simulink model "Electrical787"  (R2013a)
settings: Solver=ode45  StartTime=0.0  StopTime=MSSN.gen.time(end)  RelTol=1e-3
InitFcn:
  | load('SampleOutput.mat')
  | 
  | load('SampleFuelBurn.mat')
undefined symbols (not defined in the file): ailerons, B_737, elevator, FuelBurn, landing_gear, rudder, thrust_rev
libraries: PowerFlowLib x95, simulink x17
(part 1 of 17)
settings Model: Creator=mwillms4  LastModifiedBy=Andrew
settings DataIOCC: SignalLoggingSaveFormat=ModelDataLogs
settings OptimizationCC: ExpressionDepthLimit=2147483647
settings DebuggingCC: FcnCallInpInsideContextMsg=EnableAllAsWarning  UnconnectedInputMsg=none  UnconnectedOutputMsg=none  UnconnectedLineMsg=none
settings GRTTargetCC: CombineOutputUpdateFcns=off  GRTInterface=on

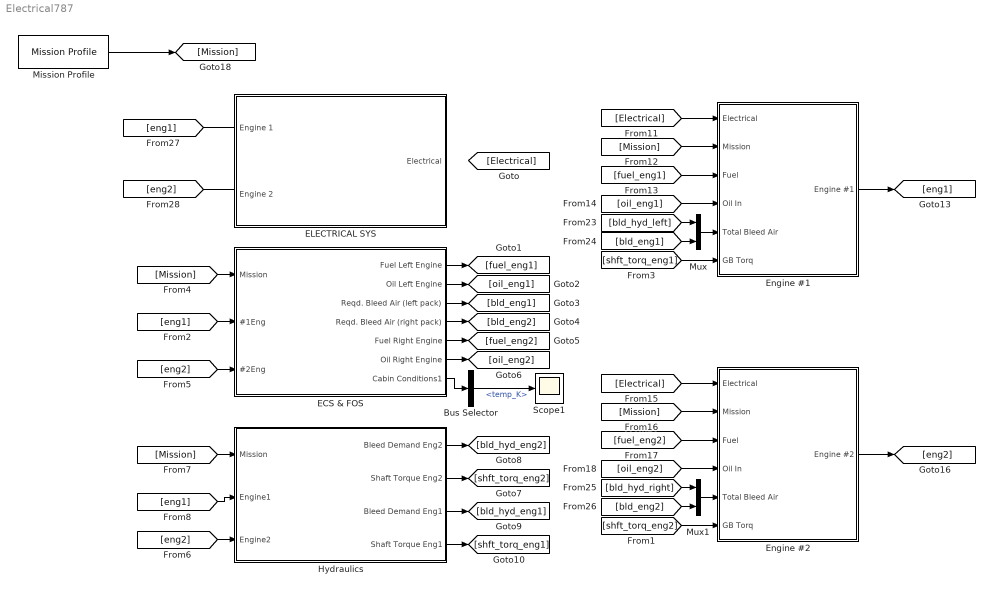
== system Electrical787 ==
  Bus Selector : BusSelector  OutputSignals=temp_K
  "ECS & FOS " : Subsystem
  "ELECTRICAL SYS " : Subsystem
  Engine #1 : Subsystem
  Engine #2 : Subsystem
  "Hydraulics " : Subsystem
  Mission Profile : PowerFlowLib/Mission Profile/Mission Profile  mssn_check=off  mssn_prof=MSSN  del_P=0  del_T=0  del_rho=0  pres_msl=101.3  temp_msl=15  dens_msl=1.229
  Mux : Mux  Inputs=2
  Mux1 : Mux  Inputs=2
  Scope1 : Scope
      settings: YMin=282  YMax=299  SaveName=ScopeData36
  wires:
  Mission Profile/1 -> [Mission]
  ? -> [Electrical]
  Engine #1/1(Engine #1) -> [eng1]
  Engine #2/1(Engine #2) -> [eng2]
  "Hydraulics "/1(Bleed Demand Eng2) -> [bld_hyd_eng2]
  "Hydraulics "/3(Bleed Demand Eng1) -> [bld_hyd_eng1]
  "ECS & FOS "/1("Fuel Left Engine ") -> [fuel_eng1]
  "ECS & FOS "/2(Oil Left Engine) -> [oil_eng1]
  "ECS & FOS "/3(Reqd. Bleed Air (left pack)) -> [bld_eng1]
  "ECS & FOS "/4(Reqd. Bleed Air (right pack)) -> [bld_eng2]
  "ECS & FOS "/5(Fuel Right Engine) -> [fuel_eng2]
  "ECS & FOS "/6(Oil Right Engine) -> [oil_eng2]
  [Mission] -> "Hydraulics "/1(Mission)
  [eng2] -> "Hydraulics "/3(Engine2)
  [eng1] -> "Hydraulics "/2(Engine1)
  [Mission] -> "ECS & FOS "/1(Mission)
  [Electrical] -> Engine #1/1(Electrical)
  [Mission] -> Engine #1/2(Mission)
  [fuel_eng1] -> Engine #1/3(Fuel)
  [oil_eng1] -> Engine #1/4(Oil In)
  [Electrical] -> Engine #2/1(Electrical)
  [Mission] -> Engine #2/2(Mission)
  [fuel_eng2] -> Engine #2/3(Fuel)
  [oil_eng2] -> Engine #2/4(Oil In)
  Mux/1 -> Engine #1/5(Total Bleed Air)
  [bld_eng1] -> Mux/2
  [bld_hyd_left] -> Mux/1
  Mux1/1 -> Engine #2/5(Total Bleed Air)
  [bld_eng2] -> Mux1/2
  [bld_hyd_right] -> Mux1/1
  Bus Selector/1 -> Scope1/1  "<temp_K>"
  [eng1] -> "ECS & FOS "/2(#1Eng)
  [eng2] -> "ECS & FOS "/3(#2Eng)
  [eng1] -> ?
  [eng2] -> ?
  "ECS & FOS "/7(Cabin Conditions1) -> Bus Selector/1
  "Hydraulics "/2(Shaft Torque Eng2) -> [shft_torq_eng2]
  "Hydraulics "/4(Shaft Torque Eng1) -> [shft_torq_eng1]
  [shft_torq_eng2] -> Engine #2/6(GB Torq)
  [shft_torq_eng1] -> Engine #1/6(GB Torq)

== system Electrical787/ECS & FOS  ==
  note: Environmental Control System
  note: Fuel & Oil System
  Mission : Inport
  #1Eng : Inport  Port=2
  #2Eng : Inport  Port=3
  #1Eng1 : InportShadow  Port=2
  #1Eng2 : InportShadow  Port=2
  #2Eng1 : InportShadow  Port=3
  #2Eng2 : InportShadow  Port=3
  Bus Creator : BusCreator  Inputs=3
  Bus Selector : BusSelector  OutputSignals=Flight parameters.temp_K,Flight parameters.Mach
  Bus Selector1 : BusSelector  OutputSignals=power_kW
  Cabin Zone : PowerFlowLib/Energy & Power Systems/Thermal/ECS/Cabin Zone  A_fuselage=320  V_cab=130.3  n_pass=176  L_shell=0.003  K_shell=1  L_insulation=0.02  K_insulation=1  L_coating=0.002  K_coating=1  Vdot_sa_pass=0.009438  q_pass=60  RAR=.25  h_outside=1  h_inside=1
  Constant : Constant  Value=50
  Constant1 : Constant  Value=1700
  Constant2 : Constant  Value=1700
  Constant{3..6} (4 alike) : Constant  Value=0
  ElectricalSink : PowerFlowLib/Support Functions//Tools/ElectricalSink  Tag=Flow  Description=TwoPhase  load_loc=Empennage  ACDC_load=AC  units=Kilowatts  unq_id=6691
  ElectricalSink1 : PowerFlowLib/Support Functions//Tools/ElectricalSink  Tag=Flow  Description=TwoPhase  load_loc=Cagobay  ACDC_load=AC  units=Kilowatts  unq_id=1878
  ElectricalSink2 : PowerFlowLib/Support Functions//Tools/ElectricalSink  Tag=Flow  Description=TwoPhase  load_loc=Cabin  ACDC_load=AC  units=Kilowatts  unq_id=3506
  ElectricalSink4 : PowerFlowLib/Support Functions//Tools/ElectricalSink  Tag=Flow  Description=TwoPhase  load_loc=Cabin  ACDC_load=DC  units=Kilowatts  unq_id=8332
  Fan1 : PowerFlowLib/Energy & Power Systems/Thermal/ECS/Fan  N_fan=1725
  Fuel Tanks/Pumps : Subsystem
  Heat Exchanger : PowerFlowLib/Energy & Power Systems/Thermal/Fuel & Oil/Heat Exchanger  fld1=Oil  fld2=Air  Tw_init=90  C_wall=60000  Tw0=90  Q0=20000  H1_0=10000  A1=0.18984  mdot1_0=1.2  Tin1_0=105  Pin1_0=101  H2_0=10000  A2=0.045127  mdot2_0=1  Tin2_0=35  Pin2_0=50
  Heat Exchanger1 : PowerFlowLib/Energy & Power Systems/Thermal/Fuel & Oil/Heat Exchanger  fld1=Oil  fld2=Air  Tw_init=90  C_wall=60000  Tw0=90  Q0=20000  H1_0=10000  A1=0.18984  mdot1_0=1.2  Tin1_0=105  Pin1_0=101  H2_0=10000  A2=0.045127  mdot2_0=1  Tin2_0=35  Pin2_0=50
  Heat Exchanger2 : PowerFlowLib/Energy & Power Systems/Thermal/Fuel & Oil/Heat Exchanger  fld1=Oil  fld2=Fuel  Tw_init=80  C_wall=60000  Tw0=80  Q0=40000  H1_0=20000  A1=0.17164  mdot1_0=1  Tin1_0=55  Pin1_0=100  H2_0=20000  A2=0.53191  mdot2_0=1.2  Tin2_0=95  Pin2_0=101
  Heat Exchanger3 : PowerFlowLib/Energy & Power Systems/Thermal/Fuel & Oil/Heat Exchanger  fld1=Fuel  fld2=Oil  Tw_init=80  C_wall=60000  Tw0=80  Q0=40000  H1_0=20000  A1=0.53191  mdot1_0=1.2  Tin1_0=95  Pin1_0=101  H2_0=20000  A2=0.17164  mdot2_0=1  Tin2_0=55  Pin2_0=100
  Left PACK : Subsystem
  Memory : Memory
  Mission1 : InportShadow
  Oil Tanks/Pumps Left Wing : Subsystem
  Oil Tanks/Pumps Left Wing1 : Subsystem
  Right PACK : Subsystem
  Thermal_sources_from Electrical_power_model1 : Subsystem
  n-intlet Mixing Junction : PowerFlowLib/Energy & Power Systems/Thermal/ECS/n-intlet Mixing Junction  no_inlets=3  d_in_1=0.1  d_in_2=0.1  d_out=0.2
  "Fuel Left Engine " : Outport
  Oil Left Engine : Outport  Port=2
  Reqd. Bleed Air (left pack) : Outport  Port=3
  Reqd. Bleed Air (right pack) : Outport  Port=4
  Fuel Right Engine : Outport  Port=5
  Oil Right Engine : Outport  Port=6
  Cabin Conditions1 : Outport  Port=7
  wires:
  Left PACK/1(Reqd. Bleed air) -> Reqd. Bleed Air (left pack)/1
  Mission/1 -> Left PACK/2(MISSION), Right PACK/2(MISSION)
  Right PACK/2(Reqd. Bleed air) -> Reqd. Bleed Air (right pack)/1
  Constant/1 -> Fuel Tanks/Pumps/1(Pamb)
  Heat Exchanger1/1 -> Heat Exchanger3/2
  Fuel Tanks/Pumps/2(Fuel Right Wing) -> Heat Exchanger3/1
  Oil Tanks/Pumps Left Wing1/1(Oil To HX) -> Heat Exchanger1/1
  Constant1/1 -> Oil Tanks/Pumps Left Wing1/1(Oil Sys Pres)
  Heat Exchanger3/1 -> Fuel Right Engine/1
  Heat Exchanger/1 -> Heat Exchanger2/1
  Oil Tanks/Pumps Left Wing/1(Oil To HX) -> Heat Exchanger/1
  Constant2/1 -> Oil Tanks/Pumps Left Wing/1(Oil Sys Pres)
  Fuel Tanks/Pumps/1(Fuel Left Wing) -> Heat Exchanger2/2
  Heat Exchanger2/2 -> "Fuel Left Engine "/1
  Heat Exchanger3/2 -> Oil Right Engine/1
  Constant3/1 -> ElectricalSink1/1, ElectricalSink2/1, ElectricalSink2/2, ElectricalSink1/2, ElectricalSink/1, ElectricalSink/2
  n-intlet Mixing Junction/1 -> Memory/1
  Mission1/1 -> Bus Selector/1
  Bus Selector/1 -> Cabin Zone/2  "<temp_K>"
  Bus Selector/2 -> Cabin Zone/3  "<Mach>"
  Thermal_sources_from Electrical_power_model1/1(Thermal Loads) -> Cabin Zone/4
  Left PACK/2(Flow Out) -> n-intlet Mixing Junction/2
  Memory/1 -> Cabin Zone/1
  #1Eng2/1 -> Oil Tanks/Pumps Left Wing/2(Flow In)
  #2Eng1/1 -> Fuel Tanks/Pumps/2(Fuel Demand Right Wing)
  #1Eng1/1 -> Fuel Tanks/Pumps/3(Fuel Demand Left Wing)
  #2Eng/1 -> Oil Tanks/Pumps Left Wing1/2(Flow In)
  #1Eng/1 -> Left PACK/1(ENGINE)
  #2Eng2/1 -> Right PACK/1(ENGINE)
  Cabin Zone/1 -> Cabin Conditions1/1, [Cabin_conditions]
  [Fan_Mixing_Jn] -> n-intlet Mixing Junction/1
  [Cabin_conditions] -> Right PACK/3(Cabin Conditions)
  [Cabin_conditions] -> Left PACK/3(Cabin Conditions)
  Right PACK/1(Flow Out) -> n-intlet Mixing Junction/3
  Bus Selector1/1 -> ElectricalSink4/1  "<power_kW>"
  Cabin Zone/2 -> Fan1/1
  Fan1/1 -> [Fan_Mixing_Jn]
  Fan1/2 -> Bus Selector1/1
  Heat Exchanger2/1 -> Oil Left Engine/1
  Bus Creator/1 -> Heat Exchanger1/2, Heat Exchanger/2
  Constant4/1 -> Bus Creator/1  "pres_kPa"
  Constant5/1 -> Bus Creator/2  "temp_K"
  Constant6/1 -> Bus Creator/3  "mdot_kgps"

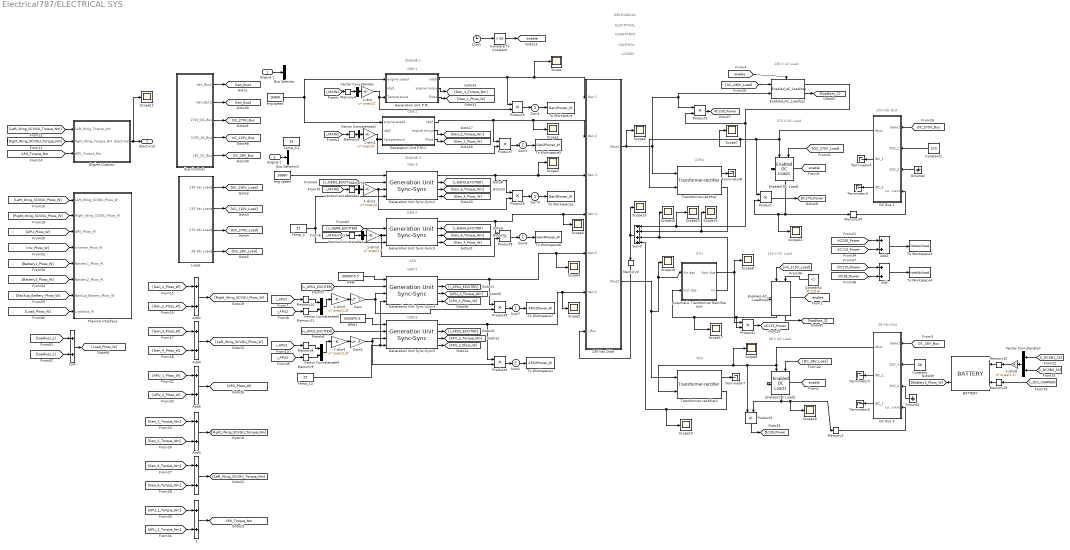
== system Electrical787/ELECTRICAL SYS  ==
  note: GEN 1
  note: ENGINE 1
  note: GEN 2
  note: GEN 3
  note: ENGINE 2
  note: GEN 4
  note: GEN 5
  note: APU
  note: GEN 6
  note: ATRU
  note: TRU
  note: 230 V AC Load
  note: 270 Vdc Dist
  note: 28 Vdc Dist
  note: 270 V DC Load
  note: CONSTANTS
  note: CONTROL
  note: LOSSES
  note: MECHANICAL
  note: ELECTRICAL
  note: ATU
  note: 115 V AC Load
  note: 28 V DC Load
  Engine 1 : Inport
  Engine 2 : Inport  Port=2
  " " : Sum
  " 1" : Sum
  1-dim{,1..3} (4 alike) : Gain  Gain=ones(1)'  Multiplication=Matrix(u*K)
  1-dim4 : Gain  Gain=ones(1,2)'  Multiplication=Matrix(u*K)
  1-dim5 : Gain  Gain=ones(1,2)'  Multiplication=Matrix(u*K)
  1-dim8 : Gain  Gain=ones(1,2)'  Multiplication=Matrix(u*K)
  230 Vac Distr : Subsystem
  Add{,1..5} (6 alike) : Sum
  Automatic Transformer Rectifier Unit : Subsystem
  BATTERY : PowerFlowLib/Energy & Power Systems/Electrical/Battery/BATTERY  NO_CELLS=9  NO_MODULES=10  INITIAL_SOC=1
  Bus Selector : BusSelector  OutputSignals=Spools.HPSpoolSpeed_rpm
  Bus Selector1 : BusSelector  OutputSignals=Spools.HPSpoolSpeed_rpm
  Bus Controls : Subsystem  mask{BUS1=Generator 1, BUS2=Generator 2, MBUS1=Generator Bus 1, ACTBUS1=Generator Bus 1, MBUS2=Generator Bus 2, ACTBUS2=Generator Bus 2, IDCBUS1=Battery 1, IDCBUS2=Battery 2}
      mask prompts: BUS1 "Source for Bus 1"; BUS2 "Source for Bus 2"; MBUS1 "Load on Main Bus 1 drawn from"; ACTBUS1 "Load on AC Transfer Bus 1 drawn from"; MBUS2 "Load on Main Bus 2 drawn from"; ACTBUS2 "Load on AC Transfer Bus 2 drawn from"; IDCBUS1 "Source for DC Service Bus 1"; IDCBUS2 "Source for DC Service Bus 2"
      mask help:
      | Specify the source from which different buses receive power. There are
      | 1. Two Generator buses (Bus 1-2)
      | 2. Two AC Main buses (Main Bus 1-2))
      | 3. Two AC Transfer buses and (AC Transfer Bus 1-2)
      | 4. Two DC Intermediate buses (DC Intermediate Bus 1-2)
      mask init:
      | switch BUS1
      |     case 1
      |         BUS1CONTROL = 1;
      |     case 2
      |         BUS1CONTROL = 2;
      |     case 3
      |         BUS1CONTROL = 3;
      |     case 4
      |         BUS1CONTROL = 4;
      | end
      | 
      | switch BUS2
      |     case 1
      |         BUS2CONTROL = 1;
      |     case 2
      |         BUS2CONTROL = 2;
      |     case 3
      |         BUS2CONTROL = 3;
      |     case 4
      |         BUS2CONTROL = 4;
      | end
      | 
      | switch MBUS1
      |     case 1
      |         MBUS1CONTROL = 1;
      |     case 2
      |         MBUS1CONTROL = 2;
      | end
      | 
      | switch ACTBUS1
      |     case 1
      |         ACTBUS1CONTROL = 1;
      |     case 2
      |         ACTBUS1CONTROL = 2;
      | end
      | 
      | switch MBUS2
      |     case 1
      |         MBUS2CONTROL = 1;
      |     case 2
      |         MBUS2CONTROL = 2;
      | end
      | 
      | switch ACTBUS2
      |     case 1
      |         ACTBUS2CONTROL = 1;
      |     case 2
      |         ACTBUS2CONTROL = 2;
      | end
      | 
      | switch IDCBUS1
      |     case 1
      |         IDCBUS1CONTROL = 1;
      |     case 2
      |         IDCBUS1CONTROL = 2;
      | end
      | 
      | switch IDCBUS2
      |     case 1
      |         IDCBUS2CONTROL = 1;
      |     case 2
      |         IDCBUS2CONTROL = 2;
      | end
      mask TypeOptions BUS1: Generator 1  | APU  | GND | AUX SUPPLY
      mask TypeOptions BUS2: Generator 2  | APU  | GND | AUX SUPPLY
      mask TypeOptions MBUS1: Generator Bus 1 | Generator Bus 2
      mask TypeOptions ACTBUS1: Generator Bus 1 | Generator Bus 2
      mask TypeOptions MBUS2: Generator Bus 1 | Generator Bus 2
      mask TypeOptions ACTBUS2: Generator Bus 1 | Generator Bus 2
      mask TypeOptions IDCBUS1: Battery 1 | Battery 2
      mask TypeOptions IDCBUS2: Battery 1 | Battery 2
  Clock : Clock
  Compare To Constant : simulink/Logic and Bit Operations/Compare To Constant  relop=>  const=50  OutDataTypeStr=uint8
  Constant : Constant  Value=28
  Constant1 : Constant  Value=270
  Constant2 : Constant  Value=[0,115,0]
  DC Bus 1 : Subsystem  mask(DC Service Bus){}
      mask help: Service Bus
  DC Bus 3 : Subsystem  mask(DC Service Bus){}
      mask help: Service Bus
  Enabled DC Load1 : PowerFlowLib/Energy & Power Systems/Electrical/Loads/Enabled  DC Load1
  Enabled DC Load2 : PowerFlowLib/Energy & Power Systems/Electrical/Loads/Enabled  DC Load1
  Enabled_AC_Loadloss : PowerFlowLib/Energy & Power Systems/Electrical/Loads/Enabled_AC_Loadloss  P=500  PF=0.85  ILRMS=0  R=10000  X=10000
  Enabled_AC_Loadloss1 : PowerFlowLib/Energy & Power Systems/Electrical/Loads/Enabled_AC_Loadloss  P=500  PF=0.85  ILRMS=0  R=10000  X=10000
  Engine Outputs : Subsystem
  Gain : Gain  Gain=.5  Multiplication=Matrix(u*K)
  Gain1 : Gain  Gain=.5  Multiplication=Matrix(u*K)
  Generation Unit P.M. : Subsystem  AncestorBlock=PowerFlowLib/Energy & Power Systems/Electrical/Systems/Generation Unit Sync-Sync  mask{machine_mode=100kVA_Gen, Rs=0.0163, Xls=0.00054, Xmd=0.66176, Xmq=0.00099, R_fd=0.016, Xlfd=0.2092, R_1d=0.2047, Xl1d=0.6524, R_1q=0.0429, R_2q=0.0429, Xl1q=0.0639, Xl2q=0.0639, ws=377, RTL=0.001, XTL=0.1, KA=20, KF=0.063, T_f=0.35, TA=0.2, KE=1, TE=0.314, SB=100000, VBDQ=100, wB=377, P=6, H=0.1777, R_conv_gen=0.05, mc_gen=10000, Vnom=230, fan_load='init_fan_characteristics.mat', exciter_param='exciter.mat'}
      mask prompts: machine_mode "Machine Preset"; Rs "Stator Resistance [ohm]"; Xls "Stator Leakage Reactance [ohm]"; Xmd "Magnetizing Direct Axis Reactance [ohm]"; Xmq "Magnetizing Quadrature Axis Reactance [ohm]"; R_fd "Field Resistance [ohm]"; Xlfd "Field Leakage Reactance [ohm]"; R_1d "Transient Direct Axis Resistance [ohm]"; Xl1d "Transient Leakage Direct Axis Reactance [ohm]"; R_1q "Transient Quadrature Axis Resistance [ohm]"; R_2q "Subtransient Quadrature Axis Resistance [ohm]"; Xl1q "Transient Leakage Quadrature Axis Reactance [ohm]"; Xl2q "Subtransient Leakage Quadrature Axis Reactance [ohm]"; ws "Rotational Speed [rad/s]"; RTL "Resistance [ohm]"; XTL "Reactance [ohm]"; SB "Baes Complex Power [VA]"; VBDQ "Base Direct and Quadrature Axis Armature Voltage [V]"; wB "Base Electrical Frequency [rad/s]"; P "Number of Pole Pairs"; H "Shaft Inertia Constant [s]"; Vnom "Nominal Voltage [V]"; fan_load "Fan Load"; exciter_param "Exciter Machine Parameters"
      mask help:
      | A generator system block implements a generic power generation unit consisting of a gearbox, a synchronous generator, a synchronous exciter and exciter controls.
      | The generator size can be selected from the drop window below.
      | (For advanced-users) When the User-defined option is selected from the drop window, the generator parameters can be manually specified in the tabs below.
      |
      | Block Inputs:
      |
      | #1: Jet engine low pressure spool [RPM]
      | #2: Exciter system supply voltage [V]
      | #3: Synchronous reference frame line currents  [A]
      |
      | Block Output:
      |
      | #1: Synchronous reference frame line voltages [V]
      | #2: Exciter system supply current [A]
      | #3: Electromagnetic torque on the low pressure spool  [N-M]
      | #4: Heat rejected to the cooling system or ambient [W]
      mask init:
      | load(fan_load);
      | 
      | % Inductances
      | Xd = Xls + Xmd;
      | Xq = Xls + Xmq;
      | Xfd = Xlfd + Xmd;
      | X1q = Xl1q + Xmq;
      | Xd1 = Xd - Xmd^2/Xfd;
      | Xq1 = Xq - Xmq^2/X1q;
      | Xd2 = Xls + (1/(1/Xmd + 1/Xlfd + 1/Xl1d));
      | Xq2 = Xls + (1/(1/Xmq + 1/Xl1q + 1/Xl2q));
      | Tdo1 = Xfd/ws/R_fd;
      | Tqo1 = X1q/ws/R_1q;
      | Tdo2 = 1/ws/R_1d*(Xl1d + 1/(1/Xmd + 1/Xlfd));
      | Tqo2 = 1/ws/R_2q*(Xl2q+1/(1/Xmq + 1/Xl1q));
      | 
      | % Base Quantities
      | 
      | TB = (P/2)*SB/wB;
      | IBDQ = SB/VBDQ;
      | LBDQ = VBDQ/wB;
      | 
      | IBFD = IBDQ;
      | IB1D = IBDQ;
      | IB1Q = IBDQ;
      | IB2Q = IBDQ;
      | 
      | VBFD = SB/IBFD;
      | VB1D = SB/IB1D;
      | VB1Q = SB/IB1Q;
      | VB2Q = SB/IB2Q;
      | 
      | LBFD = VBFD/wB;
      | LB1D = VB1D/wB;
      | LB1Q = VB1Q/wB;
      | LB2Q = VB2Q/wB;
      | 
      | J = 2*H/(wB*2/P)^2*SB;
      | M = 2*H/wB;
      | 
      | % Exciter
      | 
      | data_exc = load(exciter_param);
      |   
      | % Stator
      | Rs_exc = data_exc.r(1);
      | Xls_exc = data_exc.r(2);
      | Xmd_exc = data_exc.r(3);
      | Xmq_exc = data_exc.r(4);
      | 
      | % Field
      | R_fd_exc = data_exc.r(5);
      | Xlfd_exc = data_exc.r(6);
      | % Dampers
      | R_1d_exc = data_exc.r(7);
      | Xl1d_exc = data_exc.r(8);
      | R_1q_exc = data_exc.r(9);
      | Xl1q_exc = data_exc.r(10);
      | R_2q_exc = data_exc.r(11);
      | Xl2q_exc = data_exc.r(12);
      | 
      | % Rotor
      | P_exc = data_exc.r(13);
      | ws_exc = data_exc.r(14);
      | 
      | % Inductances
      | Xd_exc = Xls_exc + Xmd_exc;
      | Xq_exc = Xls_exc + Xmq_exc;
      | Xfd_exc = Xlfd_exc + Xmd_exc;
      | X1q_exc = Xl1q_exc + Xmq_exc;
      | Xd1_exc = Xd_exc - Xmd_exc^2/Xfd_exc;
      | Xq1_exc = Xq_exc - Xmq_exc^2/X1q_exc;
      | Xd2_exc = Xls_exc + (1/(1/Xmd_exc + 1/Xlfd_exc + 1/Xl1d_exc));
      | Xq2_exc = Xls_exc + (1/(1/Xmq_exc + 1/Xl1q_exc + 1/Xl2q_exc));
      | Tdo1_exc = Xfd_exc/ws_exc/R_fd_exc;
      | Tqo1_exc = X1q_exc/ws_exc/R_1q_exc;
      | Tdo2_exc = 1/ws_exc/R_1d_exc*(Xl1d_exc + 1/(1/Xmd_exc + 1/Xlfd_exc));
      | Tqo2_exc = 1/ws_exc/R_2q_exc*(Xl2q_exc+1/(1/Xmq_exc + 1/Xl1q_exc));
      | 
      | % Transmission Line
      | RTL_exc = data_exc.r(15);
      | XTL_exc = data_exc.r(16);
      | 
      | % Regulator and Governor
      | KA_exc = data_exc.r(17);
      | KF_exc = data_exc.r(18);
      | T_f_exc = data_exc.r(19);
      | TA_exc = data_exc.r(20);
      | KE_exc = data_exc.r(21);
      | TE_exc = data_exc.r(22);
      | 
      | % Base Quantities
      | SB_exc = data_exc.r(23);
      | VBDQ_exc = data_exc.r(24);
      | wB_exc = data_exc.r(25);
      | P_exc = data_exc.r(13);
      | H_exc = data_exc.r(26);
      | 
      | TB_exc = (P/2)*SB_exc/wB_exc;
      | IBDQ_exc = SB_exc/VBDQ_exc;
      | LBDQ_exc = VBDQ_exc/wB_exc;
      | 
      | IBFD_exc = IBDQ_exc;
      | IB1D_exc = IBDQ_exc;
      | IB1Q_exc = IBDQ_exc;
      | IB2Q_exc = IBDQ_exc;
      | 
      | VBFD_exc = SB_exc/IBFD_exc;
      | VB1D_exc = SB_exc/IB1D_exc;
      | VB1Q_exc = SB_exc/IB1Q_exc;
      | VB2Q_exc = SB_exc/IB2Q_exc;
      | 
      | LBFD_exc = VBFD_exc/wB_exc;
      | LB1D_exc = VB1D_exc/wB_exc;
      | LB1Q_exc = VB1Q_exc/wB_exc;
      | LB2Q_exc = VB2Q_exc/wB_exc;
      | 
      | J_exc = 2*data_exc.r(26)/(wB_exc*2/P_exc)^2*SB_exc;
      | M_exc = 2*H_exc/wB_exc;
      | 
      | R_conv_gen_exc = 1/data_exc.r(27);
      | mc_gen_exc = data_exc.r(28);
      mask Help: eval('open(''Generator System_help.html'')');
      mask TypeOptions machine_mode: 20kVA_Gen | 52.5kVA_Gen | 100kVA_Gen | 300kVA_Gen | 800kVA_Gen | 1MVA_Gen | User-defined
      mask Callback machine_mode:
      | h=get_param(gcb,'handle');
      | hblock=get(h);
      | data=load('GenProp.mat');
      | 
      | if strcmp(hblock.machine_mode,'User-defined')==1;
      |     adv_warn=warndlg(sprintf('User-defined parameters may lead to an unstable build.'));
      | 
      |     % grabs current values of enabled GUI parameters
      |     mskenabl = get_param(gcb,'MaskEnables');
      |     mskenabl(1:size(mskenabl,1)) = {'on'};  % sets all parameters to enable
      |     set_param(gcb,'MaskEnables',mskenabl)
      | 
      | else
      |     % For each generator preset references a column from GenProp.mat
      |     if strcmp(hblock.machine_mode,'20kVA_Gen')==1; n=1;
      |     elseif strcmp(hblock.machine_mode,'52.5kVA_Gen')==1; n=2;
      |     elseif strcmp(hblock.machine_mode,'100kVA_Gen')==1; n=3;
      |     elseif strcmp(hblock.machine_mode,'300kVA_Gen')==1; n=4;
      |     elseif strcmp(hblock.machine_mode,'800kVA_Gen')==1; n=5;
      |     elseif strcmp(hblock.machine_mode,'1MVA_Gen')==1; n=6;
      |     end
      |     % Set each parameter of the generator
      |     set1=num2str(data.r(1,n));
      |     set2=num2str(data.r(2,n));
      |     set3=num2str(data.r(3,n));
      |     set4=num2str(data.r(4,n));
      |     set_param(gcb,'Rs',set1,'Xls',set2,'Xmd',set3,'Xmq',set4)
      |     set1=num2str(data.r(5,n));
      |     set2=num2str(data.r(6,n));
      |     set_param(gcb,'R_fd',set1,'Xlfd',set2) %5 and 6
      |     set1=num2str(data.r(7,n));
      |     set2=num2str(data.r(8,n));
      |     set3=num2str(data.r(9,n));
      |     set4=num2str(data.r(10,n));
      |     set5=num2str(data.r(11,n));
      |     set6=num2str(data.r(12,n));
      |     set_param(gcb,'R_1d',set1,'Xl1d',set2,'R_1q',set3,'Xl1q',set4,'R_2q',set5,'Xl2q',set6) %7-12
      |     set1=num2str(data.r(14,n));
      |     set2=num2str(data.r(15,n));
      |     set3=num2str(data.r(16,n));
      |     set_param(gcb,'ws',set1,'RTL',set2,'XTL',set3)
      |     set1=num2str(data.r(17,n));
      |     set2=num2str(data.r(18,n));
      |     set3=num2str(data.r(19,n));
      |     set4=num2str(data.r(20,n));
      |     set5=num2str(data.r(21,n));
      |     set6=num2str(data.r(22,n));
      |     set_param(gcb,'KA',set1,'KF',set2,'T_f',set3,'TA',set4,'KE',set5,'TE',set6)
      |     set1=num2str(data.r(23,n));
      |     set2=num2str(data.r(24,n));
      |     set3=num2str(data.r(25,n));
      |     set4=num2str(data.r(13,n));
      |     set5=num2str(data.r(26,n));
      |     set_param(gcb,'SB',set1,'VBDQ',set2,'wB',set3,'P',set4,'H',set5)
      |     set1=num2str(1/data.r(27,n));
      |     set2=num2str(data.r(28,n));
      |     set_param(gcb,'R_conv_gen',set1,'mc_gen',set2)
      | 
      |     % grabs current values of enabled GUI parameters
      |     mskenabl = get_param(gcb,'MaskEnables');
      |     % sets all parameters to enable
      |     mskenabl(2:size(mskenabl,1)-3) = {'off'};
      |     set_param(gcb,'MaskEnables',mskenabl)
      | 
      | 
      | end
      | 
      | 
      | clear h hblock n data mskenabl
      | clear set1 set2 set3 set4 set5 set6
      mask Display:
      | image(imread('Generator.png')) % Load image
      | 
      | % Define inputs
      | 
      | port_label('input',1,'{\bf \omega_s_h_a_f_t}','Texmode','on')
      | port_label('input',2,'{\bf V_D_C}','Texmode','on')
      | port_label('input',3,'{\bf I_d_q_0}','Texmode','on')
      | port_label('input',4,'{\bf Temp}','Texmode','on')
      | 
      | % Define outputs
      | 
      | port_label('output',1,'{\bf V_d_q_0}','Texmode','on')
      | port_label('output',2,'{\bf I_D_C}','Texmode','on')
      | port_label('output',3,'{\bf \tau}','Texmode','on')
      | port_label('output',4,'{\bf P_l_o_s_s}','Texmode','on')
      | 
      | % % Define inputs
      | %
      | % port_label('input',1,'{\bf Generator Speed}','Texmode','on')
      | % port_label('input',2,'{\bf Battery Voltage}','Texmode','on')
      | % port_label('input',3,'{\bf Line Currents}','Texmode','on')
      | %
      | % % Define outputs
      | %
      | % port_label('output',1,'{\bf Line Voltages}','Texmode','on')
      | % port_label('output',2,'{\bf Battery Current}','Texmode','on')
      | % port_label('output',3,'{\bf Generator Torque}','Texmode','on')
      | % port_label('output',4,'{\bf Power Loss}','Texmode','on')
  Generation Unit P.M.1 : Subsystem  AncestorBlock=PowerFlowLib/Energy & Power Systems/Electrical/Systems/Generation Unit Sync-Sync  mask{machine_mode=100kVA_Gen, Rs=0.0163, Xls=0.00054, Xmd=0.66176, Xmq=0.00099, R_fd=0.016, Xlfd=0.2092, R_1d=0.2047, Xl1d=0.6524, R_1q=0.0429, R_2q=0.0429, Xl1q=0.0639, Xl2q=0.0639, ws=377, RTL=0.001, XTL=0.1, KA=20, KF=0.063, T_f=0.35, TA=0.2, KE=1, TE=0.314, SB=100000, VBDQ=100, wB=377, P=6, H=0.1777, R_conv_gen=0.05, mc_gen=10000, Vnom=230, fan_load='init_fan_characteristics.mat', exciter_param='exciter.mat'}
      mask prompts: machine_mode "Machine Preset"; Rs "Stator Resistance [ohm]"; Xls "Stator Leakage Reactance [ohm]"; Xmd "Magnetizing Direct Axis Reactance [ohm]"; Xmq "Magnetizing Quadrature Axis Reactance [ohm]"; R_fd "Field Resistance [ohm]"; Xlfd "Field Leakage Reactance [ohm]"; R_1d "Transient Direct Axis Resistance [ohm]"; Xl1d "Transient Leakage Direct Axis Reactance [ohm]"; R_1q "Transient Quadrature Axis Resistance [ohm]"; R_2q "Subtransient Quadrature Axis Resistance [ohm]"; Xl1q "Transient Leakage Quadrature Axis Reactance [ohm]"; Xl2q "Subtransient Leakage Quadrature Axis Reactance [ohm]"; ws "Rotational Speed [rad/s]"; RTL "Resistance [ohm]"; XTL "Reactance [ohm]"; SB "Baes Complex Power [VA]"; VBDQ "Base Direct and Quadrature Axis Armature Voltage [V]"; wB "Base Electrical Frequency [rad/s]"; P "Number of Pole Pairs"; H "Shaft Inertia Constant [s]"; Vnom "Nominal Voltage [V]"; fan_load "Fan Load"; exciter_param "Exciter Machine Parameters"
      mask help:
      | A generator system block implements a generic power generation unit consisting of a gearbox, a synchronous generator, a synchronous exciter and exciter controls.
      | The generator size can be selected from the drop window below.
      | (For advanced-users) When the User-defined option is selected from the drop window, the generator parameters can be manually specified in the tabs below.
      |
      | Block Inputs:
      |
      | #1: Jet engine low pressure spool [RPM]
      | #2: Exciter system supply voltage [V]
      | #3: Synchronous reference frame line currents  [A]
      |
      | Block Output:
      |
      | #1: Synchronous reference frame line voltages [V]
      | #2: Exciter system supply current [A]
      | #3: Electromagnetic torque on the low pressure spool  [N-M]
      | #4: Heat rejected to the cooling system or ambient [W]
      mask init: same as Electrical787/ELECTRICAL SYS /Generation Unit P.M.
      mask Help: eval('open(''Generator System_help.html'')');
      mask TypeOptions machine_mode: 20kVA_Gen | 52.5kVA_Gen | 100kVA_Gen | 300kVA_Gen | 800kVA_Gen | 1MVA_Gen | User-defined
      mask Callback machine_mode:
      | h=get_param(gcb,'handle');
      | hblock=get(h);
      | data=load('GenProp.mat');
      | 
      | if strcmp(hblock.machine_mode,'User-defined')==1;
      |     adv_warn=warndlg(sprintf('User-defined parameters may lead to an unstable build.'));
      | 
      |     % grabs current values of enabled GUI parameters
      |     mskenabl = get_param(gcb,'MaskEnables');
      |     mskenabl(1:size(mskenabl,1)) = {'on'};  % sets all parameters to enable
      |     set_param(gcb,'MaskEnables',mskenabl)
      | 
      | else
      |     % For each generator preset references a column from GenProp.mat
      |     if strcmp(hblock.machine_mode,'20kVA_Gen')==1; n=1;
      |     elseif strcmp(hblock.machine_mode,'52.5kVA_Gen')==1; n=2;
      |     elseif strcmp(hblock.machine_mode,'100kVA_Gen')==1; n=3;
      |     elseif strcmp(hblock.machine_mode,'300kVA_Gen')==1; n=4;
      |     elseif strcmp(hblock.machine_mode,'800kVA_Gen')==1; n=5;
      |     elseif strcmp(hblock.machine_mode,'1MVA_Gen')==1; n=6;
      |     end
      |     % Set each parameter of the generator
      |     set1=num2str(data.r(1,n));
      |     set2=num2str(data.r(2,n));
      |     set3=num2str(data.r(3,n));
      |     set4=num2str(data.r(4,n));
      |     set_param(gcb,'Rs',set1,'Xls',set2,'Xmd',set3,'Xmq',set4)
      |     set1=num2str(data.r(5,n));
      |     set2=num2str(data.r(6,n));
      |     set_param(gcb,'R_fd',set1,'Xlfd',set2) %5 and 6
      |     set1=num2str(data.r(7,n));
      |     set2=num2str(data.r(8,n));
      |     set3=num2str(data.r(9,n));
      |     set4=num2str(data.r(10,n));
      |     set5=num2str(data.r(11,n));
      |     set6=num2str(data.r(12,n));
      |     set_param(gcb,'R_1d',set1,'Xl1d',set2,'R_1q',set3,'Xl1q',set4,'R_2q',set5,'Xl2q',set6) %7-12
      |     set1=num2str(data.r(14,n));
      |     set2=num2str(data.r(15,n));
      |     set3=num2str(data.r(16,n));
      |     set_param(gcb,'ws',set1,'RTL',set2,'XTL',set3)
      |     set1=num2str(data.r(17,n));
      |     set2=num2str(data.r(18,n));
      |     set3=num2str(data.r(19,n));
      |     set4=num2str(data.r(20,n));
      |     set5=num2str(data.r(21,n));
      |     set6=num2str(data.r(22,n));
      |     set_param(gcb,'KA',set1,'KF',set2,'T_f',set3,'TA',set4,'KE',set5,'TE',set6)
      |     set1=num2str(data.r(23,n));
      |     set2=num2str(data.r(24,n));
      |     set3=num2str(data.r(25,n));
      |     set4=num2str(data.r(13,n));
      |     set5=num2str(data.r(26,n));
      |     set_param(gcb,'SB',set1,'VBDQ',set2,'wB',set3,'P',set4,'H',set5)
      |     set1=num2str(1/data.r(27,n));
      |     set2=num2str(data.r(28,n));
      |     set_param(gcb,'R_conv_gen',set1,'mc_gen',set2)
      | 
      |     % grabs current values of enabled GUI parameters
      |     mskenabl = get_param(gcb,'MaskEnables');
      |     % sets all parameters to enable
      |     mskenabl(2:size(mskenabl,1)-3) = {'off'};
      |     set_param(gcb,'MaskEnables',mskenabl)
      | 
      | 
      | end
      | 
      | 
      | clear h hblock n data mskenabl
      | clear set1 set2 set3 set4 set5 set6
      mask Display:
      | image(imread('Generator.png')) % Load image
      | 
      | % Define inputs
      | 
      | port_label('input',1,'{\bf \omega_s_h_a_f_t}','Texmode','on')
      | port_label('input',2,'{\bf V_D_C}','Texmode','on')
      | port_label('input',3,'{\bf I_d_q_0}','Texmode','on')
      | port_label('input',4,'{\bf Temp}','Texmode','on')
      | 
      | % Define outputs
      | 
      | port_label('output',1,'{\bf V_d_q_0}','Texmode','on')
      | port_label('output',2,'{\bf I_D_C}','Texmode','on')
      | port_label('output',3,'{\bf \tau}','Texmode','on')
      | port_label('output',4,'{\bf P_l_o_s_s}','Texmode','on')
      | 
      | % % Define inputs
      | %
      | % port_label('input',1,'{\bf Generator Speed}','Texmode','on')
      | % port_label('input',2,'{\bf Battery Voltage}','Texmode','on')
      | % port_label('input',3,'{\bf Line Currents}','Texmode','on')
      | %
      | % % Define outputs
      | %
      | % port_label('output',1,'{\bf Line Voltages}','Texmode','on')
      | % port_label('output',2,'{\bf Battery Current}','Texmode','on')
      | % port_label('output',3,'{\bf Generator Torque}','Texmode','on')
      | % port_label('output',4,'{\bf Power Loss}','Texmode','on')
  Generation Unit Sync-Sync{2..5} (4 alike) : PowerFlowLib/Energy & Power Systems/Electrical/Systems/Generation Unit Sync-Sync  machine_mode=100kVA_Gen  Rs=0.0163  Xls=0.00054  Xmd=0.66176  Xmq=0.00099  R_fd=0.016  Xlfd=0.2092  R_1d=0.2047  Xl1d=0.6524  R_1q=0.0429  R_2q=0.0429  Xl1q=0.0639  Xl2q=0.0639  ws=377  RTL=0.001  XTL=0.1  KA=20  KF=0.063  T_f=0.35  TA=0.2  KE=1  TE=0.314  SB=100000  VBDQ=100  wB=377  P=6  H=0.1777  R_conv_gen=0.05  mc_gen=10000  Vnom=115  fan_load='init_fan_characteristics.mat'  exciter_param='exciter.mat'
  Ground1 : Ground
  Ground2 : Ground
  Loads : Subsystem
  Memory{2..11,24,29,32} (13 alike) : Memory
  Product{,1..9} (10 alike) : Product
  RPM : Constant  Value=30000*0.5
  RPM1 : Constant  Value=30000*0.5
  Scope{,1..19} (20 alike) : Scope
      Scope settings: ShowLegends=on
      Scope1 settings: ShowLegends=on
      Scope10 settings: ShowLegends=on  SaveName=ScopeData10
      Scope11 settings: ShowLegends=on  SaveName=ScopeData11
      Scope12 settings: ShowLegends=on  SaveName=ScopeData12
      Scope13 settings: ShowLegends=on  SaveName=ScopeData13
      Scope14 settings: ShowLegends=on  SaveName=ScopeData14
      Scope15 settings: ShowLegends=on  SaveName=ScopeData15
      Scope16 settings: ShowLegends=on  SaveName=ScopeData16
      Scope17 settings: ShowLegends=on  SaveName=ScopeData17
      Scope18 settings: ShowLegends=on  SaveName=ScopeData18
      Scope19 settings: ShowLegends=on  SaveName=ScopeData19
      Scope2 settings: ShowLegends=on  SaveName=ScopeData2
      Scope3 settings: ShowLegends=on  SaveName=ScopeData3
      Scope4 settings: ShowLegends=on  SaveName=ScopeData4
      Scope5 settings: ShowLegends=on  SaveName=ScopeData5
      Scope6 settings: ShowLegends=on  SaveName=ScopeData6
      Scope7 settings: ShowLegends=on  SaveName=ScopeData7
      Scope8 settings: ShowLegends=on  SaveName=ScopeData8
      Scope9 settings: ShowLegends=on  SaveName=ScopeData9
  Sum : Sum
  Sum{1..2,4..7} (6 alike) : Sum  Inputs=+
  Sum3 : Sum  Inputs=++++
  Temp_C : Constant  Value=25
  Temp_C1 : Constant  Value=25
  Temp_C2 : Constant  Value=25
  Terminator{3..8} (6 alike) : Terminator
  Thermal Interface : Subsystem
  To Workspace : ToWorkspace  VariableName=Gen1Power_W  SampleTime=10  SaveFormat=Structure With Time
  To Workspace1 : ToWorkspace  VariableName=APU2Power_W  SampleTime=10  SaveFormat=Structure With Time
  To Workspace2 : ToWorkspace  VariableName=Gen3Power_W  SampleTime=10  SaveFormat=Structure With Time
  To Workspace3 : ToWorkspace  VariableName=totalacload  SampleTime=-1  SaveFormat=Timeseries
  To Workspace4 : ToWorkspace  VariableName=totaldcload  SampleTime=-1  SaveFormat=Timeseries
  To Workspace5 : ToWorkspace  VariableName=Gen2Power_W  SampleTime=10  SaveFormat=Structure With Time
  To Workspace6 : ToWorkspace  VariableName=Gen4Power_W  SampleTime=10  SaveFormat=Structure With Time
  To Workspace7 : ToWorkspace  VariableName=APU1Power_W  SampleTime=10  SaveFormat=Structure With Time
  Transformer-rectifier : PowerFlowLib/Energy & Power Systems/Electrical/Systems/Transformer-rectifier  pu=1
  Transformer-rectifier2 : PowerFlowLib/Energy & Power Systems/Electrical/Systems/Transformer-rectifier  pu=1
  Vector Concatenate{,1..3} (4 alike) : Concatenate  NumInputs=1  Mode=Multidimensional array  ConcatenateDimension=2
  Vector Concatenate4 : Concatenate  Mode=Multidimensional array  ConcatenateDimension=2
  Vector Concatenate5 : Concatenate  Mode=Multidimensional array  ConcatenateDimension=2
  Vector Concatenate7 : Concatenate  Mode=Multidimensional array  ConcatenateDimension=2
  eng speed : Constant  Value=16860
  "eng speed " : Constant  Value=16860
  Electrical : Outport
  tag scope: AC115_Power=global, AC230_Power=global, AC_115V_Bus=global, APU_Torque_Nm=global, DC270_Power=global, DC28_Power=global, DC_270V_Bus=global, DC_28V_Bus=global, Gen_Bus1=global, Gen_Bus2=global, enable=global
  wires:
  Generation Unit P.M./1(vdq0) -> Product5/1, Scope/1, 230 Vac Distr/1(Gen 1)
  Generation Unit P.M.1/1(vdq0) -> Product7/1, Scope1/1, 230 Vac Distr/2(Gen 2)
  Generation Unit Sync-Sync2/1 -> Product6/1, Scope2/1, 230 Vac Distr/3(Gen 3)
  Generation Unit Sync-Sync3/1 -> Product8/1, Scope3/1, 230 Vac Distr/4(Gen 4)
  Generation Unit Sync-Sync4/1 -> Product9/1, Scope4/1, 230 Vac Distr/5(Gen 5)
  Generation Unit Sync-Sync5/1 -> Product4/1, Scope5/1, 230 Vac Distr/6(Gen 6)
  230 Vac Distr/1(Vbus1) -> Scope6/1, Enabled_AC_Loadloss/2, Product3/1, Transformer-rectifier/1
  230 Vac Distr/2(Vbus2) -> Transformer-rectifier2/1, Scope10/1, Automatic Transformer Rectifier Unit/1(Vin dqo)
  [enable] -> Enabled_AC_Loadloss/Enable
  DC Bus 1/1(Vbus) -> Scope7/1, Transformer-rectifier/2, Product/1, Enabled DC Load1/1
  DC Bus 3/1(Vbus) -> Enabled DC Load2/1, Product2/1, Scope9/1, Transformer-rectifier2/2
  Enabled DC Load1/1 -> Scope12/1, Product/2, Memory24/1
  Memory24/1 -> DC Bus 1/4(Load current)
  Enabled DC Load2/1 -> Product2/2, Scope18/1, Memory2/1
  Memory2/1 -> DC Bus 3/4(Load current)
  [enable] -> Enabled DC Load1/Enable
  [enable] -> Enabled_AC_Loadloss1/Enable
  [enable] -> Enabled DC Load2/Enable
  Transformer-rectifier2/2 -> Scope19/1, Sum3/4
  Transformer-rectifier/2 -> Sum3/2, Scope15/1
  Enabled_AC_Loadloss/1 -> Product3/2, Scope14/1, Sum3/1
  Sum3/1 -> Scope13/1, Memory3/1
  Memory3/1 -> 230 Vac Distr/7(I_Bus)
  Enabled_AC_Loadloss1/1 -> Scope17/1, Automatic Transformer Rectifier Unit/2(Iout dqo), Product1/2
  Memory32/1 -> BATTERY/1
  1-dim8/1 -> Memory32/1
  [i_DCSB1_S2] -> Vector Concatenate7/1
  [i_DCSB2_S2] -> Vector Concatenate7/2
  Vector Concatenate7/1 -> 1-dim8/1
  Memory29/1 -> BATTERY/2
  [i_DC2_CHARGER] -> Memory29/1
  [AC_230V_Load] -> Enabled_AC_Loadloss/1
  Enabled_AC_Loadloss/2 -> [loadloss_1]
  Add/1 -> To Workspace4/1
  Add1/1 -> To Workspace3/1
  Enabled_AC_Loadloss1/2 -> [loadloss_2]
  [AC_115V_Load] -> Enabled_AC_Loadloss1/1
  [DC_270V_Load] -> Enabled DC Load1/2
  Loads/1(230 Vac Loads) -> [AC_230V_Load]
  Loads/2(115 Vac Loads) -> [AC_115V_Load]
  Loads/3(270 Vdc Loads) -> [DC_270V_Load]
  Loads/4(28 Vdc Loads) -> [DC_28V_Load]
  [DC_270V_Bus] -> DC Bus 1/1(Select)
  [DC_28V_Bus] -> DC Bus 3/1(Select)
  Bus Controls/1(Gen_Bus1) -> [Gen_Bus1]
  Bus Controls/2(Gen_Bus2) -> [Gen_Bus2]
  Bus Controls/5(28V_DC_Bus) -> [DC_28V_Bus]
  BATTERY/2 -> [Battery2_Ploss_W]
  Bus Controls/4(115V_AC_Bus) -> [AC_115V_Bus]
  Bus Controls/3(270V_DC_Bus) -> [DC_270V_Bus]
  [i_MAIN1] -> Memory4/1
  [i_MAIN2] -> Memory6/1
  [i_MAIN2] -> Memory7/1
  [i_MAIN1] -> Memory5/1
  Memory7/1 -> Vector Concatenate3/1
  Vector Concatenate3/1 -> 1-dim3/1
  1-dim3/1 -> Product8/2, Generation Unit Sync-Sync3/3
  Memory6/1 -> Vector Concatenate2/1
  Vector Concatenate2/1 -> 1-dim2/1
  1-dim2/1 -> Product6/2, Generation Unit Sync-Sync2/3
  Memory5/1 -> Vector Concatenate1/1
  Vector Concatenate1/1 -> 1-dim1/1
  1-dim1/1 -> Product7/2, Generation Unit P.M.1/3(Temperature)
  Memory4/1 -> Vector Concatenate/1
  Vector Concatenate/1 -> 1-dim/1
  1-dim/1 -> Generation Unit P.M./3(Temperature), Product5/2
  Clock/1 -> Compare To Constant/1
  Compare To Constant/1 -> [enable]
  Engine 2/1 -> Bus Selector1/1
  Generation Unit Sync-Sync2/2 -> [i_GEN3_EXCITER]
  Generation Unit Sync-Sync3/2 -> [i_GEN4_EXCITER]
  [v_GEN3_EXCITER] -> Generation Unit Sync-Sync2/2
  [v_GEN4_EXCITER] -> Generation Unit Sync-Sync3/2
  Temp_C/1 -> Generation Unit Sync-Sync3/4, Generation Unit Sync-Sync2/4
  Product4/1 -> Sum2/1
  Sum2/1 -> To Workspace1/1
  Vector Concatenate4/1 -> 1-dim4/1
  [i_APU2] -> Memory9/1
  [i_APU1] -> Memory8/1
  Memory8/1 -> Vector Concatenate4/1
  Memory9/1 -> Vector Concatenate4/2
  [v_APU2_EXCITER] -> Generation Unit Sync-Sync5/2
  Temp_C2/1 -> Generation Unit Sync-Sync4/4, Generation Unit Sync-Sync5/4
  Vector Concatenate5/1 -> 1-dim5/1
  [i_APU2] -> Memory11/1
  [i_APU1] -> Memory10/1
  Memory10/1 -> Vector Concatenate5/1
  Memory11/1 -> Vector Concatenate5/2
  [v_APU1_EXCITER] -> Generation Unit Sync-Sync4/2
  Product5/1 -> Sum1/1
  Sum1/1 -> To Workspace/1
  Product6/1 -> Sum4/1
  Sum4/1 -> To Workspace2/1
  Product7/1 -> Sum5/1
  Sum5/1 -> To Workspace5/1
  Product8/1 -> Sum6/1
  Sum6/1 -> To Workspace6/1
  Product9/1 -> Sum7/1
  Sum7/1 -> To Workspace7/1
  [Left_Wing_SCVGU_Torque_Nm] -> Engine Outputs/1(Left_Wing_Toqrue_Nm)
  [Right_Wing_SCVGU_Torque_Nm] -> Engine Outputs/2(Rght_Wing_Torque_Nm)
  [APU_Torque_Nm] -> Engine Outputs/3(APU_Torque_Nm)
  [Left_Wing_SCVGU_Ploss_W] -> Thermal Interface/1(Left_Wing_SCVGU_Ploss_W)
  [Right_Wing_SCVGU_Ploss_W] -> Thermal Interface/2(Right_Wing_SCVGU_Ploss_W)
  [APU_Ploss_W] -> Thermal Interface/3(APU_Ploss_W)
  [Inv_Ploss_W] -> Thermal Interface/4(Inverter_Ploss_W)
  [Battery1_Ploss_W] -> Thermal Interface/5(Battery1_Ploss_W)
  [Battery2_Ploss_W] -> Thermal Interface/6(Battery2_Ploss_W)
  [Backup_Battery_Ploss_W] -> Thermal Interface/7(Backup_Battery_Ploss_W)
  [Load_Ploss_W] -> Thermal Interface/8(Loadloss_W)
  [loadloss_1] -> Sum/1
  [loadloss_2] -> Sum/2
  Sum/1 -> [Load_Ploss_W]
  Generation Unit Sync-Sync4/3 -> [APU_1_Torque_Nm]
  Generation Unit Sync-Sync5/3 -> [APU_2_Torque_Nm]
  Generation Unit Sync-Sync4/2 -> [i_APU1_EXCITER]
  Generation Unit Sync-Sync4/4 -> [APU_1_Ploss_W]
  Generation Unit Sync-Sync5/4 -> [APU_2_Ploss_W]
  Generation Unit Sync-Sync5/2 -> [i_APU2_EXCITER]
  Generation Unit P.M./3(Ploss) -> [Gen_1_Ploss_W]
  Generation Unit P.M./2(engine torque) -> [Gen_1_Torque_Nm]
  Generation Unit P.M.1/2(engine torque) -> [Gen_2_Torque_Nm]
  Generation Unit P.M.1/3(Ploss) -> [Gen_2_Ploss_W]
  Add4/1 -> [Left_Wing_SCVGU_Ploss_W]
  Add2/1 -> [Right_Wing_SCVGU_Ploss_W]
  [Gen_1_Ploss_W] -> Add2/1
  [Gen_2_Ploss_W] -> Add2/2
  Generation Unit Sync-Sync3/4 -> [Gen_4_Ploss_W]
  Generation Unit Sync-Sync2/4 -> [Gen_3_Ploss_W]
  [Gen_4_Ploss_W] -> Add4/2
  [Gen_3_Ploss_W] -> Add4/1
  Add3/1 -> [Right_Wing_SCVGU_Torque_Nm]
  " "/1 -> [Left_Wing_SCVGU_Torque_Nm]
  Generation Unit Sync-Sync3/3 -> [Gen_4_Torque_Nm]
  Generation Unit Sync-Sync2/3 -> [Gen_3_Torque_Nm]
  [Gen_1_Torque_Nm] -> Add3/1
  [Gen_2_Torque_Nm] -> Add3/2
  [Gen_3_Torque_Nm] -> " "/1
  [Gen_4_Torque_Nm] -> " "/2
  1-dim5/1 -> Gain/1
  Gain/1 -> Product9/2, Generation Unit Sync-Sync4/3
  Gain1/1 -> Product4/2, Generation Unit Sync-Sync5/3
  1-dim4/1 -> Gain1/1
  " 1"/1 -> [APU_Torque_Nm]
  [APU_1_Torque_Nm] -> " 1"/1
  [APU_2_Torque_Nm] -> " 1"/2
  Add5/1 -> [APU_Ploss_W]
  [APU_2_Ploss_W] -> Add5/2
  [APU_1_Ploss_W] -> Add5/1
  [DC_28V_Load] -> Enabled DC Load2/2
  DC Bus 1/3(IDC_2) -> Terminator3/1
  DC Bus 1/2(IDC_1) -> Terminator4/1
  DC Bus 3/2(IDC_1) -> Terminator5/1
  DC Bus 3/3(IDC_2) -> Terminator6/1
  Transformer-rectifier2/1 -> Terminator7/1
  Transformer-rectifier/1 -> Terminator8/1
  Ground1/1 -> DC Bus 3/3(VDC_2)
  Ground2/1 -> DC Bus 1/3(VDC_2)
  RPM/1 -> Generation Unit Sync-Sync4/1
  RPM1/1 -> Generation Unit Sync-Sync5/1
  Automatic Transformer Rectifier Unit/2(Iin) -> Scope16/1, Sum3/3
  Engine Outputs/1(Electrical) -> Scope11/1, Electrical/1
  Constant1/1 -> DC Bus 1/2(VDC_1)
  Product3/1 -> [AC230_Power]
  [AC230_Power] -> Add1/1
  Product/1 -> [DC270_Power]
  Product1/1 -> [AC115_Power]
  Product2/1 -> [DC28_Power]
  [AC115_Power] -> Add1/2
  [DC270_Power] -> Add/1
  [DC28_Power] -> Add/2
  Automatic Transformer Rectifier Unit/1(Vout dqo) -> Product1/1, Scope8/1
  Constant/1 -> DC Bus 3/2(VDC_1)
  Engine 1/1 -> Bus Selector/1
  "eng speed "/1 -> Generation Unit P.M.1/1(engine speed), Generation Unit P.M./1(engine speed)
  eng speed/1 -> Generation Unit Sync-Sync2/1
  Constant2/1 -> Enabled_AC_Loadloss1/2
